simulink model "gnc_ministack_v2"  (R2025a)
settings: Solver=VariableStepAuto  StartTime=0.0  StopTime=60  RelTol=1e-3
undefined symbols (not defined in the file): config
libraries: sim3dlib x1, aerolibsim3d x1
settings Model: SimulationMode=accelerator  Creator=Jackt  LastModifiedBy=Jackt

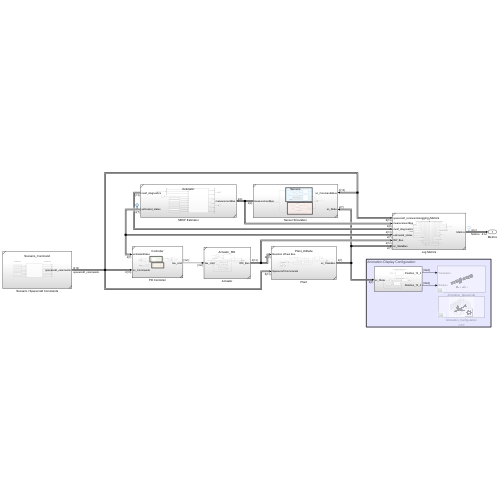
[thumbnail: Simulink's stored preview of the top-level diagram]
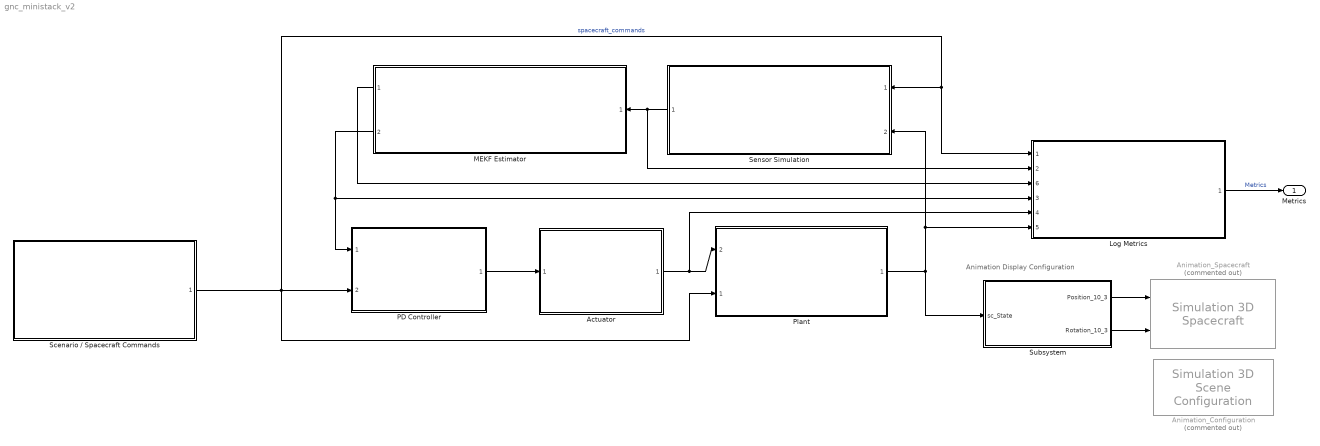
== system gnc_ministack_v2 ==
  note: Animation Display Configuration
  Actuator : Subsystem  ReferencedSubsystem=Actuator_RW
  Animation_Configuration : sim3dlib/Simulation 3D Scene Configuration  Priority=0  Commented=on  ProjectFormat=Default Scenes  SceneDesc=Earth  ProjectName=C:\Program Files\MATLAB\R2025a\toolbox\shared\sim3d_projects\automotive_project_windows\UE\WindowsNoEditor\VehicleSimulation.exe  ScenePath=/Game/Maps/HwStrght  EnableOpenDRIVE=off  vehTagList={'Custom';'Scene Origin';'SimulinkVehicle1'}  vehTag=SimulinkVehicle1  AttachedCameraRelativeTranslation=[0 0 0]  FreeCameraDefaultInitialTranslation=[-14000000, 0, 0]  AttachedCameraRelativeRotation=[0 0 0]  FreeCameraDefaultInitialRotation=[0, 0, 0]  ViewpointName=Custom  FreeCameraInitialTranslation=[-6, 0, 2]  ViewpointTranslation=[0 0 0]  FreeCameraInitialRotation=[0, -15, 0]  ViewpointRotation=[0 0 0]  OpVisEn=off  Ts=.02  EnableWindow=on  EnableRemoteAccess=off  EnableWeather=on  SunAzimuth=205.200  SunAltitude=40.0  EnableGeospatialSun=off  Latitude=0  Longitude=0  Date=2023-01-01  Time=10:30:00  GeoTimeZone=-5.0  SunDaylightSaving=off  wind=1  clouds=10  EnableVolumetricClouds=off  CloudCoverage=0  CloudAltitude=6  fog=0  rain=0  RaindropsEffect=off  SnowDensity=0  EnableGeospatial=off  TilesetSource=Earth terrain  UseTrueOrigin=off  OriginHeight=200  OriginLatitude=40.744652  OriginLongitude=-73.988864  MapStyle=Aerial  AdditionalAssetIDs=[]  UseAdvancedSunSky=off  SolarTime=11  TimeZone=-5  Day=21  Month=9  Year=2022  UseDaylightSavingTime=on  DSTStartDay=10  DSTStartMonth=3  DSTEndDay=3  DSTEndMonth=11  DSTSwitchHour=2  sensorTag=MainCamera1  sensorId=1  sensorName=MainCamera1  mountLoc=Origin  offsetFlag=off  tmountOffset=[0, 0, 0]  rmountOffset=[0, 0, 0]  HorizontalResolution=1280  VerticalResolution=720  HorizontalFOV=60  mountPoint=[0 0 0]  mountOrientation=[0 0 0]  aMode=0  ID=1  GeoTrigger=Inactive  ViewNameList={'Custom'}  ViewTranslationList={'[-6 0 2]'}  ViewRotationList={'[0 -15 0]'}
      settings: AttributesFormatString=ICRF  LibrarySourceBlock=aerolibsim3d/Simulation 3D Scene Configuration
  Animation_Spacecraft : aerolibsim3d/Simulation 3D Spacecraft  Priority=-1  Commented=on  Mesh=CubeSat  MeshPath=/MathWorksAerospaceContent/Vehicles/Spacecraft/CubeSat/Mesh/SK_CubeSat.SK_CubeSat  MeshPathSmall=/MathWorksAerospaceContent/Vehicles/Spacecraft/SmallSat/Mesh/SK_SmallSat.SK_SmallSat  SpacecraftColor=Silver  ActorName=SimulinkVehicle1  Translation=zeros(10, 3)  Rotation=zeros(10, 3)  ScaleInputPort=Dialog  Scale=[1 1 1]  InitialScale=[1 1 1]  IsGHSensorEnabled=off  AreGHRaysVisible=off  IsOutputReshapeEnabled=on  GHRayLength=1524  GHBodyOffset=1  GHContactLocation1=[0 0 0]  GHContactLocation2=[0 0 0]  GHContactLocation3=[0 0 0]  GHContactLocation4=[0 0 0]  WoWSensorTolerance=0.05  SampleTime=-1  ActorType=SimulinkVehicle  ID=1  aMode=0  ActorTag=SimulinkVehicle1
  Log Metrics : Subsystem  ReferencedSubsystem=Logging_Metrics
      settings: PortSchema="{\"entries\":[{\"content\":{\"sides\":[{\"content\":{\"connectorIds\":[\"In1\",\"In2\",\"In6\",\"In3\",\"In4\",\"In5\"]},\"type\":\"ConnectorPlacement.EquallySpacedRectSide\",\"uuid\":\"3d1c444d-ba8e-405e-b8a8-600d7ed71bb6\"},{\"content\":{\"connectorIds\":[\"Out1\"],\"side\":\"RIGHT\"},\"type\":\"ConnectorPlacement.EquallySpacedRectSide\",\"uuid\":\"f8c84752-bea5-4192-b240-bef4b9625199\"},{\"content\":{\"side\":\"TOP\"},\"type\":\"ConnectorPlacement.EquallySpacedRectSide\",\"uuid\":\"c1466d31-89c3-4c42-bd8f-ae97f3b82410\"}]},\"type\":\"ConnectorPlacement.EquallySpacedConnector\",\"uuid\":\"a4537d45-f46a-46b5-baec-10d9d397b07c\"}],\"packageUris\":[\"http://schema.mathworks.com/mf0/Connector/R2020b\"],\"version\":\"1.0\"}"
  MEKF Estimator : Subsystem  ReferencedSubsystem=Estimator
  PD Controller : Subsystem  ReferencedSubsystem=Controller
  Plant : Subsystem  ReferencedSubsystem=Plant_Attitude
      settings: PortSchema="{\"entries\":[{\"content\":{\"sides\":[{\"content\":{\"connectorIds\":[\"In2\",\"In1\"]},\"type\":\"ConnectorPlacement.EquallySpacedRectSide\",\"uuid\":\"b2b0e650-ed80-4d3a-b2e6-cb8c771423dc\"},{\"content\":{\"connectorIds\":[\"Out1\"],\"side\":\"RIGHT\"},\"type\":\"ConnectorPlacement.EquallySpacedRectSide\",\"uuid\":\"33da7a04-3718-43bd-b08b-b0008a120dfb\"},{\"content\":{\"side\":\"TOP\"},\"type\":\"ConnectorPlacement.EquallySpacedRectSide\",\"uuid\":\"983c145a-f7c0-43d4-9f5e-34c8e2659ec7\"}]},\"type\":\"ConnectorPlacement.EquallySpacedConnector\",\"uuid\":\"481068ae-a74f-4297-8863-3095c906541d\"}],\"packageUris\":[\"http://schema.mathworks.com/mf0/Connector/R2020b\"],\"version\":\"1.0\"}"
  Scenario / Spacecraft Commands : Subsystem  ReferencedSubsystem=Scenario_Command
  Sensor Simulation : Subsystem  ReferencedSubsystem=Sensors
  Subsystem : Subsystem
  Metrics : Outport
  wires:
  Scenario / Spacecraft Commands/1 -> Sensor Simulation/1, Log Metrics/1, PD Controller/2, Plant/1  "spacecraft_commands"
  Sensor Simulation/1 -> Log Metrics/2, MEKF Estimator/1
  MEKF Estimator/2 -> PD Controller/1, Log Metrics/3
  PD Controller/1 -> Actuator/1
  Actuator/1 -> Log Metrics/4, Plant/2
  Plant/1 -> Sensor Simulation/2, Log Metrics/5, Subsystem/1(sc_State)
  Subsystem/1(Position_10_3) -> Animation_Spacecraft/1
  Subsystem/2(Rotation_10_3) -> Animation_Spacecraft/2
  MEKF Estimator/1 -> Log Metrics/6
  Log Metrics/1 -> Metrics/1  "Metrics"

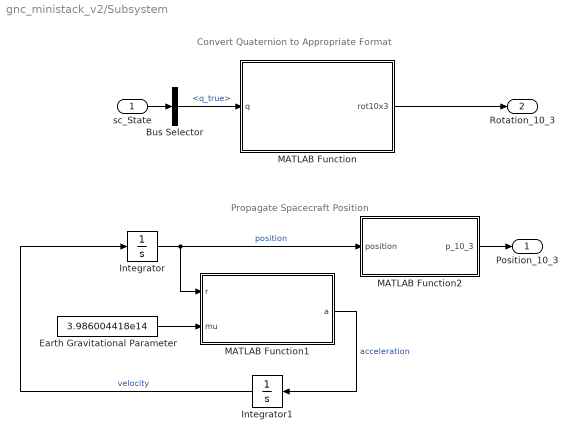
== system gnc_ministack_v2/Subsystem ==
  note: Propagate Spacecraft Position
  note: Convert Quaternion to Appropriate Format
  sc_State : Inport  OutDataTypeStr=Bus: sc_stateBus
  Bus Selector : BusSelector  OutputSignals=q_true
  Earth Gravitational Parameter : Constant  Value=3.986004418e14  VectorParams1D=off
  Integrator : Integrator  InitialCondition=config.ic.x_0
  Integrator1 : Integrator  InitialCondition=config.ic.v_0
  MATLAB Function : MATLAB Function  TreatAsAtomicUnit=on
  MATLAB Function1 : MATLAB Function  TreatAsAtomicUnit=on
  MATLAB Function2 : MATLAB Function  TreatAsAtomicUnit=on
  Position_10_3 : Outport
  Rotation_10_3 : Outport  Port=2
  wires:
  MATLAB Function/1(rot10x3) -> Rotation_10_3/1
  Integrator/1 -> MATLAB Function1/1(r), MATLAB Function2/1(position)  "position"
  MATLAB Function1/1(a) -> Integrator1/1  "acceleration"
  MATLAB Function2/1(p_10_3) -> Position_10_3/1
  Integrator1/1 -> Integrator/1  "velocity"
  Earth Gravitational Parameter/1 -> MATLAB Function1/2(mu)
  sc_State/1 -> Bus Selector/1
  Bus Selector/1 -> MATLAB Function/1(q)  "<q_true>"

== matlab function gnc_ministack_v2/Subsystem/MATLAB Function1 ==
  data: r input; a output; mu input
function a = twoBodyAccel(r, mu)
rn = norm(r); %Calculate Radius Magnitude

%Calculate Acceleration Vector
a  = -mu * r / (rn^3); % m/s^2 
end

== matlab function gnc_ministack_v2/Subsystem/MATLAB Function2 ==
  data: position input; p_10_3 output
function p_10_3 = make_10x3(position)
    %Pre-allocate output matrix zeros
    p_10_3 = zeros(10, 3);

    %Add to output matrix
    p_10_3(1, :) = position(:)';
end

== matlab function gnc_ministack_v2/Subsystem/MATLAB Function ==
  data: q input; rot10x3 output
function rot10x3 = pack_cubesat_rpy(q)
% q: [4x1] scalar-first quaternion (assumed unit-ish)
% rot10x3: [10x3] rows are bones; row1 is BODY [roll pitch yaw] rad

q = q(:);
q = q / max(norm(q), 1e-12);

% Optional: stabilize sign to reduce visual "flips"
if q(1) < 0
    q = -q;
end

% Convert quaternion -> roll/pitch/yaw (ZYX yaw-pitch-roll)
q0=q(1); q1=q(2); q2=q(3); q3=q(4);

% yaw (psi)
psi = atan2(2*(q0*q3 + q1*q2), 1 - 2*(q2^2 + q3^2));
% pitch (theta)
s = 2*(q0*q2 - q3*q1);
s = min(max(s, -1), 1);
theta = asin(s);
% roll (phi)
phi = atan2(2*(q0*q1 + q2*q3), 1 - 2*(q1^2 + q2^2));

rot10x3 = zeros(10,3);
rot10x3(1,:) = [phi, theta, psi];
end
